simulink model "bacteria_population"  (R2020a)
settings: Solver=VariableStepAuto  StartTime=0.0  StopTime=1  RelTol=1e-3
settings Model: Creator=Dhanush Wagle  LastModifiedBy=Dhanush Wagle

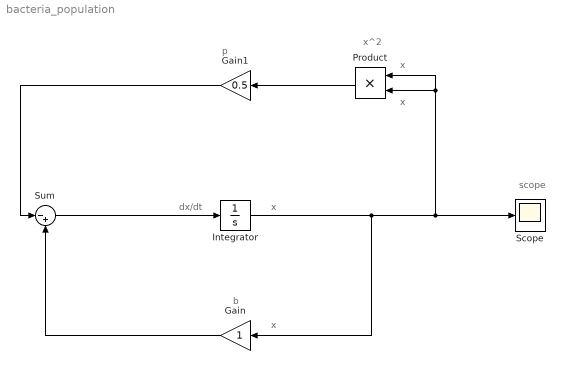
== system bacteria_population ==
  note: scope
  note: x^2
  note: dx/dt
  note: x
  note: p
  note: b
  note: x
  note: x
  note: x
  Gain : Gain
  Gain1 : Gain  Gain=0.5
  Integrator : Integrator  InitialCondition=100
  Product : Product
  Scope : Scope
  Sum : Sum  Inputs=|-+
  wires:
  Integrator/1 -> Gain/1, Product/1, Product/2, Scope/1
  Gain/1 -> Sum/2
  Gain1/1 -> Sum/1
  Sum/1 -> Integrator/1
  Product/1 -> Gain1/1
